simulink model "modelo"  (Simulink 10.3)
settings: Solver=ode45  StartTime=0.0  StopTime=10.0  RelTol=1e-3  EnableMultiTasking=on
undefined symbols (not defined in the file): q1, q2, q3, r1
settings Model: Creator=Guillermo  LastModifiedBy=feder
settings DataIOCC: LimitDataPoints=on
settings OptimizationCC: InitFltsAndDblsToZero=on
settings DebuggingCC: SaveWithParameterizedLinksMsg=none  SignalResolutionControl=TryResolveAllWithWarning  SolverPrmCheckMsg=warning  MultiTaskDSMMsg=warning  MultiTaskCondExecSysMsg=none
settings GRTTargetCC: TargetFcnLib=ansi_tfl_tmw.mat

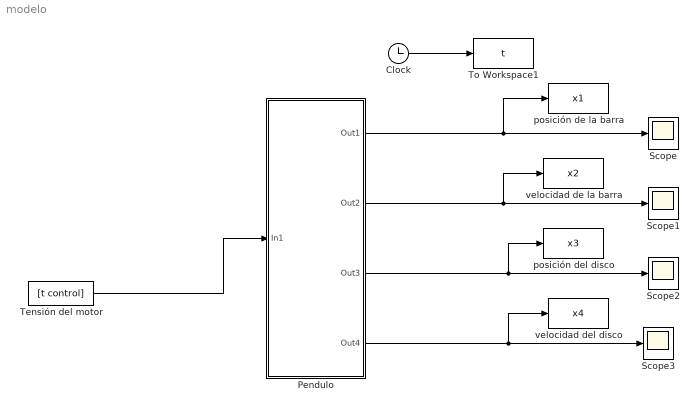
== system modelo ==
  Clock : Clock
  Pendulo : Subsystem
  Scope{,1..3} (4 alike) : Scope
  Tensión del motor : FromWorkspace  VariableName=[t control]  SampleTime=0.01  ZeroCross=off
  To Workspace1 : ToWorkspace  VariableName=t  SampleTime=-1
  posición de la barra : ToWorkspace  VariableName=x1  SampleTime=-1
  posición del disco : ToWorkspace  VariableName=x3  SampleTime=-1
  velocidad de la barra : ToWorkspace  VariableName=x2  SampleTime=-1
  velocidad del disco : ToWorkspace  VariableName=x4  SampleTime=-1
  wires:
  Clock/1 -> To Workspace1/1
  Pendulo/1(Out1) -> Scope/1, posición de la barra/1
  Pendulo/2(Out2) -> velocidad de la barra/1, Scope1/1
  Pendulo/3(Out3) -> posición del disco/1, Scope2/1
  Pendulo/4(Out4) -> velocidad del disco/1, Scope3/1
  Tensión del motor/1 -> Pendulo/1(In1)

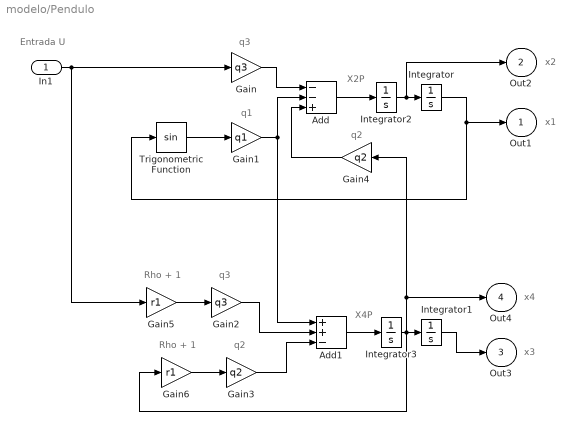
== system modelo/Pendulo ==
  note: x4
  note: x3
  note: x1
  note: x2
  note: X2P
  note: q1
  note: q3
  note: Entrada U
  note: q2
  note: q3
  note: Rho + 1
  note: q2
  note: Rho + 1
  note: X4P
  In1 : Inport
  Add : Sum  Inputs=--+
  Add1 : Sum  Inputs=++-
  Gain : Gain  Gain=q3
  Gain1 : Gain  Gain=q1
  Gain2 : Gain  Gain=q3
  Gain3 : Gain  Gain=q2
  Gain4 : Gain  Gain=q2
  Gain5 : Gain  Gain=r1
  Gain6 : Gain  Gain=r1
  Integrator{,1..3} (4 alike) : Integrator
  Trigonometric Function : Trigonometry
  Out1 : Outport
  Out2 : Outport  Port=2
  Out3 : Outport  Port=3
  Out4 : Outport  Port=4
  wires:
  Trigonometric Function/1 -> Gain1/1
  Gain1/1 -> Add1/1, Add/2
  Add/1 -> Integrator2/1
  Gain/1 -> Add/1
  In1/1 -> Gain/1, Gain5/1
  Add1/1 -> Integrator3/1
  Gain2/1 -> Add1/2
  Integrator/1 -> Out1/1, Trigonometric Function/1
  Integrator2/1 -> Out2/1, Integrator/1
  Gain4/1 -> Add/3
  Gain5/1 -> Gain2/1
  Gain6/1 -> Gain3/1
  Integrator1/1 -> Out3/1
  Gain3/1 -> Add1/3
  Integrator3/1 -> Gain6/1, Integrator1/1, Gain4/1, Out4/1
